simulink model "LinearEQTNSimulink"  (Simulink 7.0)
settings: Solver=ode45  StartTime=0.0  StopTime=10.0  RelTol=1e-3
settings Model: Creator=Ben Favour  LastModifiedBy=Ben Favour

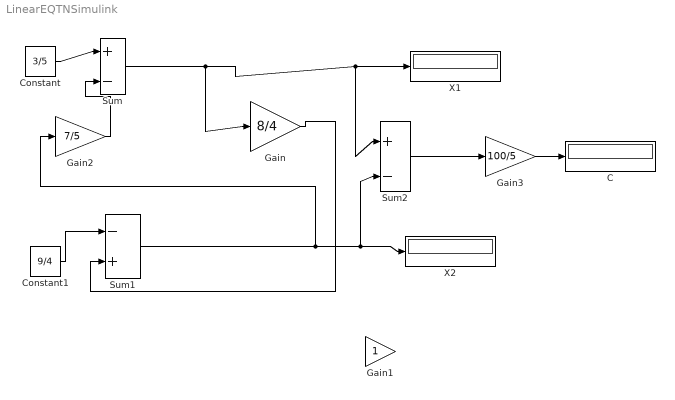
== system LinearEQTNSimulink ==
  C : Display
  Constant : Constant  Value=3/5  OutDataType=sfix(16)  OutScaling=2^0
  Constant1 : Constant  Value=9/4  OutDataType=sfix(16)  OutScaling=2^0
  Gain : Gain  Gain=8/4  ParameterDataType=sfix(16)  ParameterScaling=2^0  OutDataType=sfix(16)  OutScaling=2^0
  Gain1 : Gain  ParameterDataType=sfix(16)  ParameterScaling=2^0  OutDataType=sfix(16)  OutScaling=2^0
  Gain2 : Gain  Gain=7/5  ParameterDataType=sfix(16)  ParameterScaling=2^0  OutDataType=sfix(16)  OutScaling=2^0
  Gain3 : Gain  Gain=100/5  ParameterDataType=sfix(16)  ParameterScaling=2^0  OutDataType=sfix(16)  OutScaling=2^0
  Sum : Sum  Inputs=|+-  OutDataType=sfix(16)  OutScaling=2^0
  Sum1 : Sum  Inputs=|-+  OutDataType=sfix(16)  OutScaling=2^0
  Sum2 : Sum  Inputs=|+-  OutDataType=sfix(16)  OutScaling=2^0
  X1 : Display
  X2 : Display
  wires:
  Constant/1 -> Sum/1
  Sum/1 -> Gain/1, X1/1, Sum2/1
  Constant1/1 -> Sum1/1
  Sum1/1 -> Gain2/1, X2/1, Sum2/2
  Gain2/1 -> Sum/2
  Gain/1 -> Sum1/2
  Sum2/1 -> Gain3/1
  Gain3/1 -> C/1
